simulink model "RASS"  (R2024b)
settings: Solver=FixedStepAuto  StartTime=0.0  StopTime=150  FixedStep=0.00001  RelTol=1e-3
values from neighbouring files (symbols this model uses):
  A = [0, 1, 0, 0; -k_s/m_s, -c_s/m_s, k_s/m_s, c_s/m_s; 0, 0, 0, 1; k_s/m_u, c_s/m_u, (-k_s-k_t)/m_u, (-c_s-c_t)/m_u]    [RASS_parameters.m]
  B = [0, 0; 0, 1/m_s; 0, 0; 1/m_u, -1/m_u]    [RASS_parameters.m]
  C = [-k_s/m_s, -c_s/m_s, k_s/m_s, c_s/m_s; 0, 1, 0, 0; 0, 0, 0, 1]    [RASS_parameters.m]
  D = [0, 1/m_s; 0, 0; 0, 0]    [RASS_parameters.m]
  n = 0.94    [RASS_parameters.m]
libraries: slpidlib x1
settings Model: Creator=Mikael  LastModifiedBy=ASUS
settings RTWCC: GPUComputeCapability=3.5

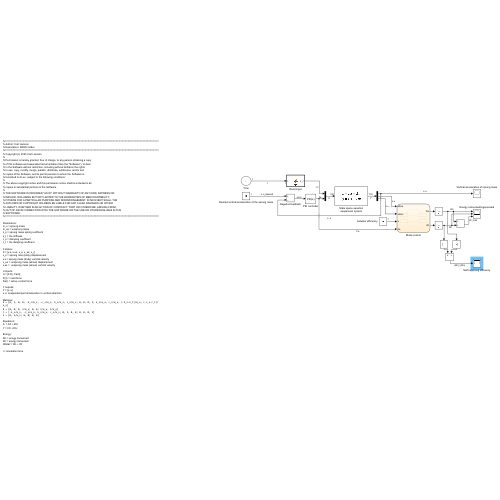
[thumbnail: Simulink's stored preview of the top-level diagram]
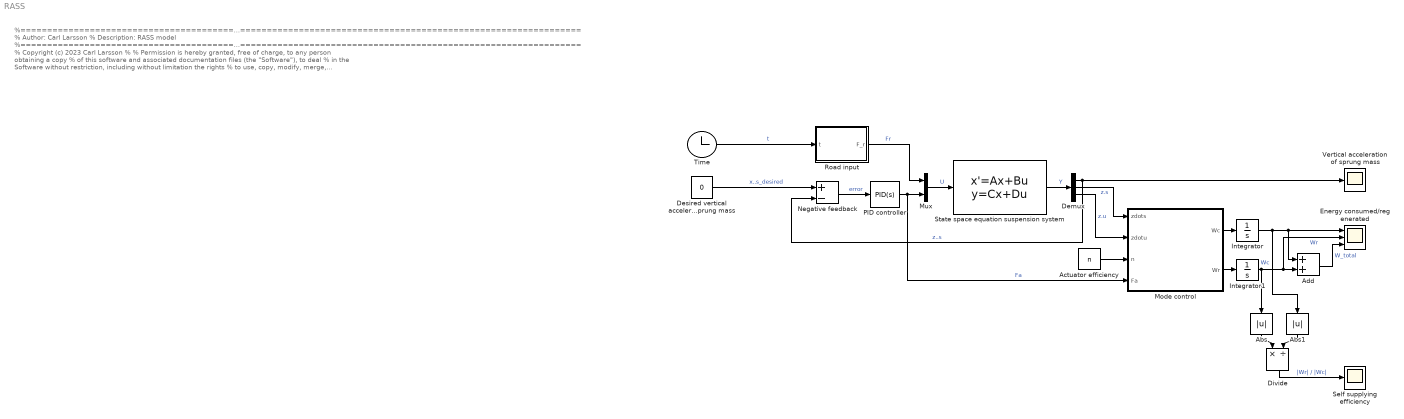
== system RASS ==
  note: %========================================================================================================
      | % Author: Carl Larsson
      | % Description: RASS model
      | %========================================================================================================
      | % Copyright (c) 2023 Carl Larsson
      | %
      | % Permission is hereby granted, free of charge, to any person obtaining a copy
      | % of this software and associated documentation files (the "Software"), to deal
      | % in the Software without restriction, including without limitation the rights
      | % to use, copy, modify, merge, publish, distribute, sublicense, and/or sell
      | % copies of the Software, and to permit persons to whom the Software is
      | % furnished to do so, subject to the following conditions:
      | %
      | % The above copyright notice and this permission notice shall be included in all
      | % copies or substantial portions of the Software.
      | %
      | % THE SOFTWARE IS PROVIDED "AS IS", WITHOUT WARRANTY OF ANY KIND, EXPRESS OR
      | % IMPLIED, INCLUDING BUT NOT LIMITED TO THE WARRANTIES OF MERCHANTABILITY,
      | % FITNESS FOR A PARTICULAR PURPOSE AND NONINFRINGEMENT. IN NO EVENT SHALL THE
      | % AUTHORS OR COPYRIGHT HOLDERS BE LIABLE FOR ANY CLAIM, DAMAGES OR OTHER
      | % LIABILITY, WHETHER IN AN ACTION OF CONTRACT, TORT OR OTHERWISE, ARISING FROM,
      | % OUT OF OR IN CONNECTION WITH THE SOFTWARE OR THE USE OR OTHER DEALINGS IN THE
      | % SOFTWARE. %========================================================================================================
      |
      | Parameters:
      | m_s = sprung mass
      | m_us = unsprung mass
      | k_s = sprung mass spring coefficent
      | k_t = tire stiffness
      | c_s = damping coefficent
      | c_t = tire damping coefficent
      |
      | X states:
      | X = [x.s, x.us, x_s, x_us, x_r]
      | x_s = sprung mas (body) displacement
      | x.s = sprung mass (body) vertical velocity
      | x_us = unsprung mass (wheel) displacement
      | x.us = unsprung mass (wheel) vertical velocity
      |
      | U inputs:
      | U = [Fr(t), Fa(t)]
      | Fr(t) = road force
      | Fa(t) = active control force
      |
      | Y outputs:
      | Y = [x..s]
      | x..s: suspended part acceleration in vertical direction
      |
      | Matrices:
      | A = [0, 1, 0, 0; -k_s/m_s, -c_s/m_s, k_s/m_s, c_s/m_s; 0, 0, 0, 1; k_s/m_u, c_s/m_u, (-k_s-k_t)/m_u, (-c_s-c_t)/m_u]
      | B = [0, 0; 0, 1/m_s; 0, 0; 1/m_u, 1/m_u]
      | C = [-k_s/m_s, -c_s/m_s, k_s/m_s, c_s/m_s; 0, 1, 0, 0; 0, 0, 0, 1]
      | D = [0, 1/m_s; 0, 0; 0, 0]
      |
      | Equations:
      | X. = AX + BU
      | Y = CX + DU
      |
      | Energy:
      | Wc = enegy consumed
      | Wr = energy harvested
      | Wtotal = Wc + Wr
      |
      | t = simulation time
  Abs : Abs  SaturateOnIntegerOverflow=off
  Abs1 : Abs  SaturateOnIntegerOverflow=off
  Actuator efficiency : Constant  Value=n
  Add : Sum
  Demux : Demux  Outputs=3
  Desired vertical acceleration of the sprung mass : Constant  Value=0
  Divide : Product  Inputs=*/
  Energy consumed/regenerated : Scope  NumInputPorts=3
  Integrator : Integrator
  Integrator1 : Integrator
  Mode control : Stateflow chart  TreatAsAtomicUnit=on
      settings: PortSchema="{\"entries\":[{\"content\":{\"sides\":[{\"content\":{\"connectorIds\":[\"In1\",\"In2\",\"In4\",\"In3\"]},\"type\":\"ConnectorPlacement.EquallySpacedRectSide\",\"uuid\":\"5ebe2246-e20d-4949-8e65-fc1642e01fd4\"},{\"content\":{\"connectorIds\":[\"Out1\",\"Out2\"],\"side\":\"RIGHT\"},\"type\":\"ConnectorPlacement.EquallySpacedRectSide\",\"uuid\":\"40acab74-05d3-4822-b3ff-804df959f27b\"},{\"content\":{\"side\":\"TOP\"},\"type\":\"ConnectorPlacement.EquallySpacedRectSide\",\"uuid\":\"6b8b2662-28ee-4ff8-bff3-bc2998b6869a\"}]},\"type\":\"ConnectorPlacement.EquallySpacedConnector\",\"uuid\":\"3ffe1391-de77-42ba-879a-09017edfc053\"}],\"packageUris\":[\"http://schema.mathworks.com/mf0/Connector/R2020b\"],\"version\":\"1.0\"}"
  Mux : Mux  Inputs=2
  Negative feedback : Sum  Inputs=+-
  PID controller : slpidlib/PID Controller  Controller=PID  Form=Parallel  TimeDomain=Continuous-time  UseExternalTs=off  SampleTime=-1  IntegratorMethod=Forward Euler  FilterMethod=Forward Euler  ControllerParametersSource=internal  P=500  I=5  UseKiTs=off  D=1  UseExternalDerivativeSource=off  N=100  UseFilter=on  TunerSelectOption=Transfer Function Based (PID Tuner App)  InitialConditionSource=internal  InitialConditionForIntegrator=0  InitialConditionForFilter=0  DifferentiatorICPrevScaledInput=0  ExternalReset=none  TrackingMode=off  Kt=1  LimitOutput=off  SatLimitsSource=internal  UpperSaturationLimit=inf  LowerSaturationLimit=-inf  LinearizeAsGain=on  AntiWindupMode=none  Kb=1  LimitIntegrator=off  UpperIntegratorSaturationLimit=inf  LowerIntegratorSaturationLimit=-inf  POutMin=[]  POutMax=[]  IOutMin=[]  IOutMax=[]  DOutMin=[]  DOutMax=[]  NOutMin=[]  NOutMax=[]  SumOutMin=[]  SumOutMax=[]  SaturationOutMin=[]  SaturationOutMax=[]  PParamMin=[]  PParamMax=[]  IParamMin=[]  IParamMax=[]  DParamMin=[]  DParamMax=[]  NParamMin=[]  NParamMax=[]  KbParamMin=[]  KbParamMax=[]  KtParamMin=[]  KtParamMax=[]  KbOutMin=[]  KbOutMax=[]  KtOutMin=[]  KtOutMax=[]  IntegratorOutMin=[]  IntegratorOutMax=[]  FilterOutMin=[]  FilterOutMax=[]  SumI1OutMin=[]  SumI1OutMax=[]  SumI2OutMin=[]  SumI2OutMax=[]  SumI3OutMin=[]  SumI3OutMax=[]  SumI4OutMin=[]  SumI4OutMax=[]  SumDOutMin=[]  SumDOutMax=[]  DifferentiatorOutMin=[]  DifferentiatorOutMax=[]  FilterDiffOutCoefMin=[]  FilterDiffOutCoefMax=[]  ReciprocalOutMin=[]  ReciprocalOutMax=[]  SumDenOutMin=[]  SumDenOutMax=[]  SumNumOutMin=[]  SumNumOutMax=[]  DivideOutMin=[]  DivideOutMax=[]  UdiffTsProdOutMin=[]  UdiffTsProdOutMax=[]  NTsProdOutMin=[]  NTsProdOutMax=[]  UintegralTsProdOutMin=[]  UintegralTsProdOutMax=[]  UngainTsProdOutMin=[]  UngainTsProdOutMax=[]  ClampingZeroOutDataTypeStr=Inherit: Inherit via back propagation  ClampingZeroOutMin=[]  ClampingZeroOutMax=[]  FilterDenConstantOutDataTypeStr=Inherit: Inherit via back propagation  FilterDenConstantOutMin=[]  FilterDenConstantOutMax=[]  PCopyOutDataTypeStr=Inherit: Inherit via back propagation  PCopyOutMin=[]  PCopyOutMax=[]  NCopyOutDataTypeStr=Inherit: Inherit via back propagation  NCopyOutMin=[]  NCopyOutMax=[]  IntegratorContinuousStateAttributes=''  IntegratorStateMustResolveToSignalObject=off  IntegratorRTWStateStorageClass=Auto  FilterContinuousStateAttributes=''  FilterStateMustResolveToSignalObject=off  FilterRTWStateStorageClass=Auto  ParallelPVariant=InternalParameters  IdealPVariant=Disabled  IVariant=InternalParameters  DVariant=InternalParameters  IntegratorVariant=Continuous  SatVariant=Disabled  AWVariant=Passthrough  PCopyVariant=Disabled  TRVariant=Disabled  FdbkBlocksVariant=Forward  IdealPFdbkVariant=Disabled  SatFdbkVariant=Disabled  DerivativeFilterVariant=ContFilter  NVariant=InternalParameters  NCopyVariant=Disabled  FilterICVariant=InternalICsFilter  IntegratorICVariant=InternalICs  ExternalResetVariant=Disabled  TRSumVariant=Passthrough  SumFdbkVariant=Disabled  SumVariant=Sum_PID  TsampFilterVariant=InternalTs  TsampNgainVariant=Passthrough  TsampIntegralVariant=Disabled_SignalSpec  ExternalSaturationOutDataTypeStr=Inherit: Same as second input  DerivativeSourceVariant=ErrorSignal  PreIntVariant=InternalPreInt
  Road input : MATLAB Function  TreatAsAtomicUnit=on
  Self supplying efficiency : Scope
  State space equation suspension system : StateSpace  A=A  B=B  C=C  D=D  InitialCondition=0
  Time : Clock
  Vertical acceleration of sprung mass : Scope
  wires:
  PID controller/1 -> Mux/2, Mode control/3(Fa)  "Fa"
  Negative feedback/1 -> PID controller/1  "error"
  Desired vertical acceleration of the sprung mass/1 -> Negative feedback/1  "x..s_desired"
  Mux/1 -> State space equation suspension system/1  "U"
  Road input/1(F_r) -> Mux/1  "Fr"
  Time/1 -> Road input/1(t)  "t"
  State space equation suspension system/1 -> Demux/1  "Y"
  Demux/1 -> Vertical acceleration of sprung mass/1, Negative feedback/2  "z..s"
  Demux/2 -> Mode control/1(zdots)  "z.s"
  Demux/3 -> Mode control/2(zdotu)  "z.u"
  Actuator efficiency/1 -> Mode control/4(n)
  Add/1 -> Energy consumed/regenerated/3  "W_total"
  Mode control/1(Wc) -> Integrator/1
  Mode control/2(Wr) -> Integrator1/1
  Integrator1/1 -> Add/2, Energy consumed/regenerated/2, Abs/1  "Wr"
  Integrator/1 -> Add/1, Energy consumed/regenerated/1, Abs1/1  "Wc"
  Divide/1 -> Self supplying efficiency/1  "|Wr| / |Wc|"
  Abs/1 -> Divide/1
  Abs1/1 -> Divide/2

== matlab function RASS/Road input ==
  settings: updateMethod=DISCRETE
  data: t input; F_r output
function F_r = fcn(t)
F_r = road_input(t);

== stateflow chart RASS/Mode control ==
  note: Mode control
  note: Actuator mode
      | Wc <= 0
  note: Generator mode
      | Wr >= 0
  state during_
    Wc = - ((Fa / n) * (zdots-zdotu));
    exit:
    Wc = 0;
  state during_1
    Wr = n * Fa * (zdots-zdotu);
    exit:
    Wr = 0;
  state during_2
    Wc =  (Fa / n) * (zdots-zdotu);
    exit:
    Wc = 0;
  state during_3
    Wr = - (n * Fa * (zdots-zdotu));
    exit:
    Wr = 0;
  during_ -> during_1 [order 1] : [(zdots-zdotu)<=0]
  (default) -> during_ : {Wc = 0;
      | Wr = 0;}
  during_1 -> during_ [order 1] : [(zdots-zdotu)>0]
  during_2 -> during_ [order 2] : [Fa>=0]
  during_ -> during_2 [order 2] : [Fa<0]
  during_1 -> during_3 [order 2] : [Fa>0]
  during_3 -> during_1 [order 2] : [Fa<=0]
  during_3 -> during_2 [order 1] : [(zdots-zdotu)>0]
  during_2 -> during_3 [order 1] : [(zdots-zdotu)<=0]
  data: zdots input; zdotu input; Wc output; Wr output; Fa input; n input
